simulink model "Simulink Model"  (R2022a)
settings: Solver=VariableStepAuto  StartTime=0.0  StopTime=60  RelTol=1e-3
libraries: slpidlib x1
settings Model: Creator=jamesbond  LastModifiedBy=jamesbond

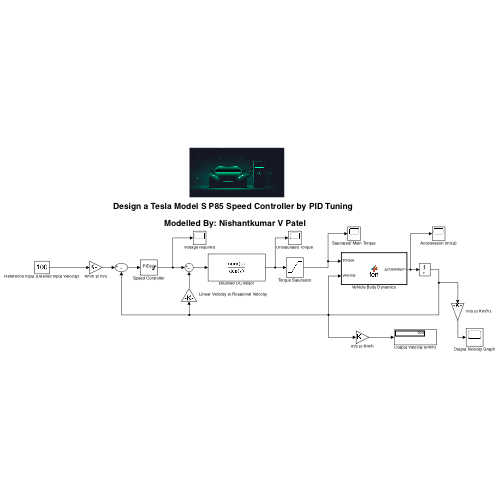
[thumbnail: Simulink's stored preview of the top-level diagram]
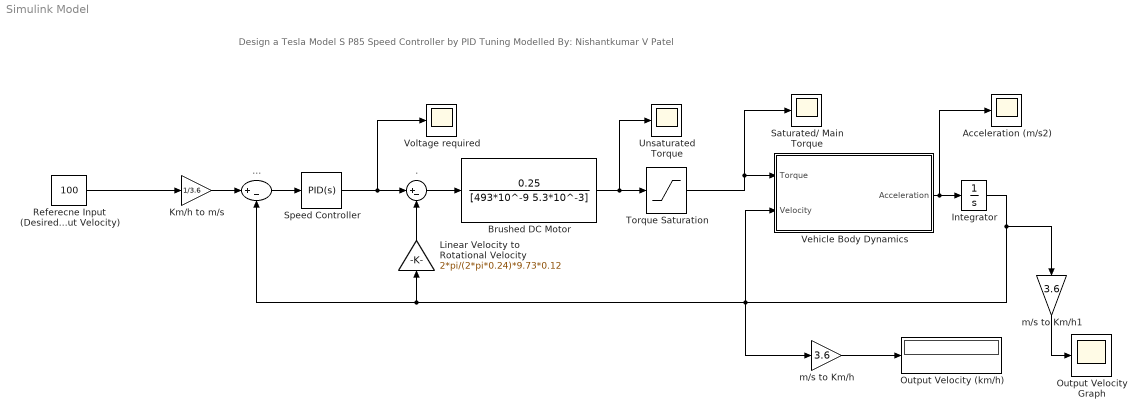
== system Simulink Model ==
  note: Design a Tesla Model S P85 Speed Controller by PID Tuning
      |
      | Modelled By: Nishantkumar V Patel
  . : Sum  Inputs=|+-
  ... : Sum  Inputs=|+-
  Acceleration (m/s2) : Scope
  Brushed DC Motor : TransferFcn  Numerator=[0.25]  Denominator=[493*10^-9 5.3*10^-3]
  Integrator : Integrator
  Km/h to m/s : Gain  Gain=1/3.6
  "Linear Velocity to Rotational Velocity " : Gain  Gain=2*pi/(2*pi*0.24)*9.73*0.12
  Output Velocity (km/h) : Display
  Output Velocity Graph : Scope
  Referecne Input (Desired Input Velocity) : Constant  Value=100
  Saturated/ Main Torque : Scope
  Speed Controller : slpidlib/PID Controller  Controller=PID  Form=Parallel  TimeDomain=Continuous-time  UseExternalTs=off  SampleTime=-1  IntegratorMethod=Forward Euler  FilterMethod=Forward Euler  ControllerParametersSource=internal  P=1500  I=300  UseKiTs=off  D=75  N=100  UseFilter=on  TunerSelectOption=Transfer Function Based (PID Tuner App)  InitialConditionSource=internal  InitialConditionForIntegrator=0  InitialConditionForFilter=0  DifferentiatorICPrevScaledInput=0  ExternalReset=none  TrackingMode=off  Kt=1  LimitOutput=on  SatLimitsSource=internal  UpperSaturationLimit=346  LowerSaturationLimit=0  LinearizeAsGain=on  AntiWindupMode=clamping  Kb=1  POutMin=[]  POutMax=[]  IOutMin=[]  IOutMax=[]  DOutMin=[]  DOutMax=[]  NOutMin=[]  NOutMax=[]  SumOutMin=[]  SumOutMax=[]  SaturationOutMin=[]  SaturationOutMax=[]  PParamMin=[]  PParamMax=[]  IParamMin=[]  IParamMax=[]  DParamMin=[]  DParamMax=[]  NParamMin=[]  NParamMax=[]  KbParamMin=[]  KbParamMax=[]  KtParamMin=[]  KtParamMax=[]  KbOutMin=[]  KbOutMax=[]  KtOutMin=[]  KtOutMax=[]  IntegratorOutMin=[]  IntegratorOutMax=[]  FilterOutMin=[]  FilterOutMax=[]  SumI1OutMin=[]  SumI1OutMax=[]  SumI2OutMin=[]  SumI2OutMax=[]  SumI3OutMin=[]  SumI3OutMax=[]  SumI4OutMin=[]  SumI4OutMax=[]  SumDOutMin=[]  SumDOutMax=[]  DifferentiatorOutMin=[]  DifferentiatorOutMax=[]  FilterDiffOutCoefMin=[]  FilterDiffOutCoefMax=[]  ReciprocalOutMin=[]  ReciprocalOutMax=[]  SumDenOutMin=[]  SumDenOutMax=[]  SumNumOutMin=[]  SumNumOutMax=[]  DivideOutMin=[]  DivideOutMax=[]  UdiffTsProdOutMin=[]  UdiffTsProdOutMax=[]  NTsProdOutMin=[]  NTsProdOutMax=[]  UintegralTsProdOutMin=[]  UintegralTsProdOutMax=[]  UngainTsProdOutMin=[]  UngainTsProdOutMax=[]  IntegratorContinuousStateAttributes=''  IntegratorStateMustResolveToSignalObject=off  IntegratorRTWStateStorageClass=Auto  FilterContinuousStateAttributes=''  FilterStateMustResolveToSignalObject=off  FilterRTWStateStorageClass=Auto  ParallelPVariant=InternalParameters  IdealPVariant=Disabled  IVariant=InternalParameters  DVariant=InternalParameters  IntegratorVariant=Continuous  SatVariant=Enabled  AWVariant=ContClampingParallel  PCopyVariant=Disabled  TRVariant=Disabled  FdbkBlocksVariant=Forward  IdealPFdbkVariant=Disabled  SatFdbkVariant=Disabled  DerivativeFilterVariant=ContFilter  NVariant=InternalParameters  NCopyVariant=Disabled  FilterICVariant=InternalICsFilter  IntegratorICVariant=InternalICs  ExternalResetVariant=Disabled  TRSumVariant=Passthrough  SumFdbkVariant=Disabled  SumVariant=Sum_PID  TsampFilterVariant=InternalTs  TsampNgainVariant=Passthrough  TsampIntegralVariant=Passthrough  ExternalSaturationOutDataTypeStr=Inherit: Same as second input  aMode=0
  Torque Saturation : Saturate  UpperLimit=600  LowerLimit=0
  Unsaturated Torque : Scope
  Vehicle Body Dynamics : MATLAB Function  TreatAsAtomicUnit=on
  Voltage required : Scope
  m/s to Km/h : Gain  Gain=3.6
  m/s to Km/h1 : Gain  Gain=3.6
  wires:
  "Linear Velocity to Rotational Velocity "/1 -> ./2
  Vehicle Body Dynamics/1(Acceleration) -> Acceleration (m/s2)/1, Integrator/1
  Integrator/1 -> m/s to Km/h/1, .../2, "Linear Velocity to Rotational Velocity "/1, Vehicle Body Dynamics/2(Velocity), m/s to Km/h1/1
  Referecne Input (Desired Input Velocity)/1 -> Km/h to m/s/1
  ./1 -> Brushed DC Motor/1
  Brushed DC Motor/1 -> Torque Saturation/1, Unsaturated Torque/1
  m/s to Km/h/1 -> Output Velocity (km/h)/1
  Torque Saturation/1 -> Saturated/ Main Torque/1, Vehicle Body Dynamics/1(Torque)
  Speed Controller/1 -> ./1, Voltage required/1
  Km/h to m/s/1 -> .../1
  .../1 -> Speed Controller/1
  m/s to Km/h1/1 -> Output Velocity Graph/1

== matlab function Simulink Model/Vehicle Body Dynamics ==
  data: Torque input; Acceleration output; Velocity input
function Acceleration = fcn(Torque, Velocity)
Acceleration=(0.6*40.54*Torque-427.7-0.3381*Velocity^2)/2180;
